simulink library "franka_simulink"  (R2025a)
settings: Solver=ode45  StartTime=0.0  StopTime=10.0  RelTol=1e-3  EnableMultiTasking=on
undefined symbols (not defined in the file or in its folder): franka_setup_bus
settings Model: Creator=vasi_ko  LastModifiedBy=kvasios
settings SolverCC: AlgebraicLoopSolver=TrustRegion
settings DataIOCC: LimitDataPoints=on  SaveFormat=Array  ReturnWorkspaceOutputs=off
settings OptimizationCC: LifeSpan=inf
settings DebuggingCC: SolverPrmCheckMsg=warning  UnconnectedInputMsg=warning  UnconnectedOutputMsg=warning  UnconnectedLineMsg=warning  SFUnexpectedBacktrackingDiag=warning  SFNoUnconditionalDefaultTransitionDiag=warning  SFExecutionAtInitializationDiag=none  ArithmeticOperatorsInVariantConditions=warning
settings HardwareCC: ProdBitPerPointer=32.0  ProdBitPerSizeT=32.0  ProdBitPerPtrDiffT=32.0  ProdLargestAtomicFloat=None  ProdIntDivRoundTo=Undefined  ProdEndianess=Unspecified  ProdWordSize=32.0  ProdHWDeviceType=32-bit Generic
settings ModelReferenceCC: EnableRefExpFcnMdlSchedulingChecks=on  PropagateSignalLabelsOutOfModel=off
settings SFSimCC: SimUseLocalCustomCode=off  CustomCodeUndefinedFunction=UseInterfaceOnly
settings RTWCC: PostCodeGenCommand=setBuildArgs(buildInfo)  RTWUseLocalCustomCode=off  GPUComputeCapability=3.5  DLArmComputeVersion=19.05
settings CodeAppCC: StateflowObjectComments=on
settings GRTTargetCC: TargetLangStandard=C89/C90 (ANSI)
settings ConfigComp: CovMetricSettings=dw  CovSaveCumulativeToWorkspaceVar=on  CovSaveSingleToWorkspaceVar=on  CovExternalEMLEnable=off  CovSFcnEnable=off

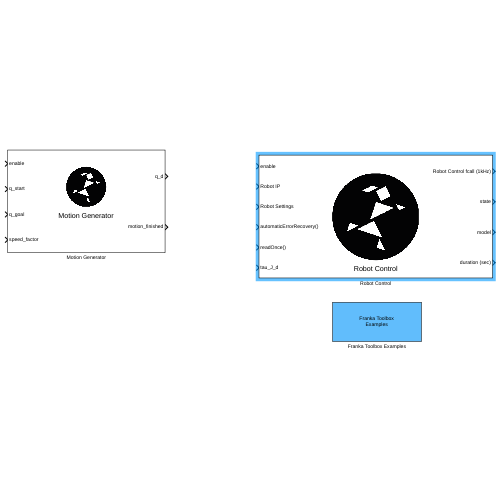
[thumbnail: Simulink's stored preview of the top-level diagram]
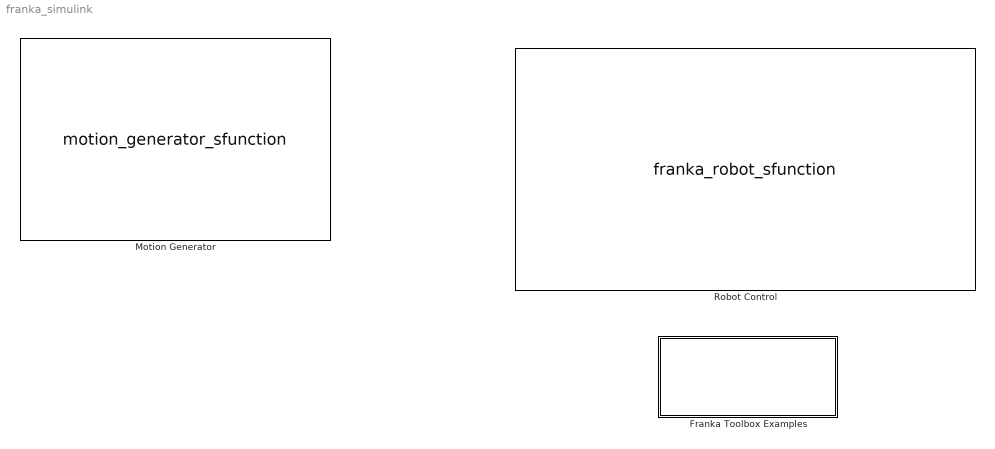
== system franka_simulink ==
  Franka Toolbox Examples : Subsystem
      settings: OpenFcn=franka_toolbox_examples;
      mask Display: disp('Franka Toolbox\nExamples')
  Motion Generator : S-Function  FunctionName=motion_generator_sfunction  SFunctionDeploymentMode=off  EnableBusSupport=off
      mask DialogControl DescTextVar Prompt: <b>Joint Motion Generator</b><br><br> Generates smooth synchronized joint-space trajectories using polynomial profiles.<br><br> <b>Inputs:</b> <ul> <li><tt>enable</tt> – Rising edge triggers motion</li> <li><tt>q_start</tt> – Start positions [rad] (7×1)</li> <li><tt>q_goal</tt> – Goal positions [rad] (7×1)</li> <li><tt>speed_factor</tt> – Speed scaling (0,1]</li> </ul> <b>Outputs:</b> <ul> <li><tt>q_d</tt> – Desired positions [rad] (7×1)</li> <li><tt>motion_finished</tt> – 1 when complete</li> </ul> All joints synchronized to finish simultaneously.
      mask Display:
      | %https://www.mathworks.com/help/simulink/slref/image.html
      | %https://www.mathworks.com/help/simulink/slref/text.html
      | 
      | % Read image
      | imagePath = fullfile(franka_installation_path_get,'data','images','franka_robotics_logo.png');
      | pic = imread(imagePath);
      | 
      | % Block size (Simulink canvas units)
      | pos = get_param(gcb,'Position');  % [left top right bottom]
      | block_w = pos(3) - pos(1);
      | block_h = pos(4) - pos(2);
      | 
      | % ---- Layout (reserve space at bottom for text) ----
      | text_band_h = 0.25 * block_h;    % bottom band for label
      | gap         = 0.04 * block_h;    % gap between label and image area
      | img_area_y0 = text_band_h + gap; % image area starts above text+gap
      | img_area_h  = block_h - img_area_y0;
      | 
      | % ---- Scale image down more ----
      | img_h = size(pic,1);
      | img_w = size(pic,2);
      | 
      | max_w = 0.55 * block_w;          % smaller than your 0.60
      | max_h = 0.55 * img_area_h;
      | 
      | scale  = min(max_w/img_w, max_h/img_h);
      | draw_w = img_w * scale;
      | draw_h = img_h * scale;
      | 
      | % Center image in the upper (image) area
      | x_img = (block_w - draw_w) / 2;
      | y_img = img_area_y0 + (img_area_h - draw_h) / 2;
      | 
      | image(pic, [x_img y_img draw_w draw_h]);
      | 
      | % Text centered in the bottom band
      | x_txt = block_w/2;
      | y_txt = text_band_h + text_band_h/2;
      | 
      | text(x_txt, y_txt, '{\fontsize{14}Motion Generator}', ...
      |      HorizontalAlignment='center', ...
      |      VerticalAlignment='middle', ...
      |      texmode='on');
      | 
      | port_label('input',1,'enable');
      | port_label('input',2,'q_start');
      | port_label('input',3,'q_goal');
      | port_label('input',4,'speed_factor');
      | 
      | port_label('output',1,'q_d');
      | port_label('output',2,'motion_finished');
  Robot Control : S-Function  LoadFcn=franka_setup_bus();  FunctionName=franka_robot_sfunction  Parameters=control_mode  SFunctionDeploymentMode=off  EnableBusSupport=off  mask{control_mode=Torques}
      mask prompts: control_mode "Control Mode Select:"
      mask DialogControl franka_robot_block_description Prompt: <b>Franka Robot Control</b><br></br>Real-time interface to the Franka Robot via libfranka. Executes the connected function-call subsystem synchronously within the robot's 1kHz control loop.<br><br>  <b>Control Modes:</b> Torques, JointPositions, JointVelocities, CartesianPose, CartesianVelocities (single-callback), or Torques + motion generator (dual-callback).<br><br>  <b>Inputs:</b><br> • <i>Enable</i> – Rising edge applies settings and starts control; falling edge stops gracefully<br> • <i>robot_ip</i> – Robot IP address (16-char ASCII)<br> • <i>settings</i> – FrankaRobotSettingsBus (impedance, collision thresholds, EE frames, load)<br> • <i>error_recovery</i> – Rising edge triggers automatic error recovery (when not in control)<br> • <i>read_once</i> – Rising edge reads robot state once (when not in control)<br> • <i>command</i> – Control command (mode-dependent)<br><br>  <b>Outputs:</b><br> • <i>fcall</i> – Function-call trigger at 1kHz<br> • <i>robot_state</i> – FrankaRobotStateBus (complete robot state)<br> • <i>model_data</i> – FrankaModelDataBus (M, c, g, J)<br> • <i>dt</i> – Control period [s]
      mask Display:
      | %https://www.mathworks.com/help/simulink/slref/image.html
      | % Read image
      | imagePath = fullfile(franka_installation_path_get,'data','images','franka_robotics_logo.png');
      | pic = imread(imagePath);
      | 
      | % Block size (pixels)
      | pos = get_param(gcb,'Position');  % [left top right bottom]
      | block_w = pos(3) - pos(1);
      | block_h = pos(4) - pos(2);
      | 
      | % ---- Layout: keep your icon sizing, just reserve space for text ----
      | text_band_h = 0.25 * block_h;     % space for label at bottom
      | gap         = 0.04 * block_h;     % gap between image and text
      | img_area_y0 = text_band_h + gap;
      | img_area_h  = block_h - img_area_y0;
      | 
      | % Image native size
      | img_h = size(pic,1);
      | img_w = size(pic,2);
      | 
      | % Keep your existing icon scaling (0.60) but apply it to the IMAGE AREA
      | max_w = 1 * block_w;
      | max_h = 1 * img_area_h;
      | 
      | % Scale without distortion
      | scale  = min(max_w/img_w, max_h/img_h);
      | draw_w = img_w * scale;
      | draw_h = img_h * scale;
      | 
      | % Center image in the upper image area
      | x_img = (block_w - draw_w) / 2;
      | y_img = img_area_y0 / 2 + (img_area_h - draw_h) / 2;
      | 
      | % Draw image
      | image(pic, [x_img y_img draw_w draw_h]);
      | 
      | % Draw text underneath
      | x_txt = block_w/2;
      | y_txt = text_band_h/3;
      | 
      | text(x_txt, y_txt, '{\fontsize{14}Robot Control}', ...
      |      HorizontalAlignment='center', ...
      |      VerticalAlignment='middle', ...
      |      texmode='on');
      | 
      | port_label('input',1,'enable');
      | port_label('input',2,'Robot IP');
      | port_label('input',3,'Robot Settings');
      | port_label('input',4,'automaticErrorRecovery()');
      | port_label('input',5,'readOnce()');
      | 
      | control_mode = get_param(gcb, 'control_mode');
      | 
      | switch control_mode
      |     % ====================================================================
      |     % Single-callback modes (0-4)
      |     % ====================================================================
      |     case 'Torques'
      |         % Port 5: tau_J_d (7)
      |         port_label('input', 6, 'tau_J_d');
      | 
      |     case 'Joint Positions'
      |         % Port 5: q_d (7)
      |         port_label('input', 6, 'q_d');
      | 
      |     case 'Joint Velocities'
      |         % Port 5: dq_d (7)
      |         port_label('input', 6, 'dq_d');
      | 
      |     case 'Cartesian Pose'
      |         % Port 5: O_T_EE_d (16), Port 6: elbow_d (2)
      |         port_label('input', 6, 'O_T_EE_d');
      |         port_label('input', 7, 'elbow_d');
      | 
      |     case 'Cartesian Velocities'
      |         % Port 5: O_dP_EE_d (6), Port 6: elbow_d (2)
      |         port_label('input', 6, 'O_dP_EE_d');
      |         port_label('input', 7, 'elbow_d');
      | 
      |     % ====================================================================
      |     % Dual-callback modes (5-8): Torque + Motion Generator
      |     % ====================================================================
      |     case 'Torques + Joint Positions'
      |         % Port 5: tau_J_d (7), Port 6: q_d (7)
      |         port_label('input', 6, 'tau_J_d');
      |         port_label('input', 7, 'q_d');
      | 
      |     case 'Torques + Joint Velocities'
      |         % Port 5: tau_J_d (7), Port 6: dq_d (7)
      |         port_label('input', 6, 'tau_J_d');
      |         port_label('input', 7, 'dq_d');
      | 
      |     case 'Torques + Cartesian Pose'
      |         % Port 5: tau_J_d (7), Port 6: O_T_EE_d (16), Port 7: elbow_d (2)
      |         port_label('input', 6, 'tau_J_d');
      |         port_label('input', 7, 'O_T_EE_d');
      |         port_label('input', 8, 'elbow_d');
      | 
      |     case 'Torques + Cartesian Velocities'
      |         % Port 5: tau_J_d (7), Port 6: O_dP_EE_d (6), Port 7: elbow_d (2)
      |         port_label('input', 6, 'tau_J_d');
      |         port_label('input', 7, 'O_dP_EE_d');
      |         port_label('input', 8, 'elbow_d');
      | end
      | 
      | port_label('output',1,'Robot Control fcall (1kHz)');
      | port_label('output',2,'state');
      | port_label('output',3,'model');
      | port_label('output',4,'duration (sec)');

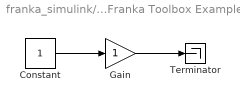
== system franka_simulink/Franka Toolbox Examples ==
  Constant : Constant
  Gain : Gain
  Terminator : Terminator
  wires:
  Constant/1 -> Gain/1
  Gain/1 -> Terminator/1
